simulink model "FusionMODEL_version1"  (R2018a)
settings: Solver=FixedStepAuto  StartTime=0.0  StopTime=SimulationTime  FixedStep=SamplingTime  RelTol=1e-3
undefined symbols (not defined in the file or in its folder): ACTIVATE_CAM, ACTIVATE_RAD, CAM1_detTimeStamp, CAM1_MeasNoise, CAM1_objClassID, CAM1_PX, CAM1_PY, CAM1_VX, CAM1_VY, CAM2_detTimeStamp, CAM2_MeasNoise, CAM2_objClassID, CAM2_PX, CAM2_PY, CAM2_VX, CAM2_VY, CAM3_detTimeStamp, CAM3_MeasNoise, CAM3_objClassID, CAM3_PX, CAM3_PY, CAM3_VX, CAM3_VY, CAM4_detTimeStamp, CAM4_MeasNoise, CAM4_objClassID, CAM4_PX, CAM4_PY, CAM4_VX, CAM4_VY, CAM5_detTimeStamp, CAM5_MeasNoise, CAM5_objClassID, CAM5_PX, CAM5_PY, CAM5_VX, CAM5_VY, CAM6_detTimeStamp, CAM6_MeasNoise, CAM6_objClassID, CAM6_PX, CAM6_PY, CAM6_VX, CAM6_VY, CAM7_detTimeStamp, CAM7_MeasNoise, CAM7_objClassID, CAM7_PX, CAM7_PY, CAM7_VX, CAM7_VY, CAM8_detTimeStamp, CAM8_MeasNoise, CAM8_objClassID, CAM8_PX, CAM8_PY, CAM8_VX, CAM8_VY, CAM_nMeas, CAM_TYPE ... (+151)
libraries: simulink_extras x2
(part 1 of 6)
settings Model: SimulationMode=accelerator  Creator=Udit Bhaskar  LastModifiedBy=Udit Bhaskar

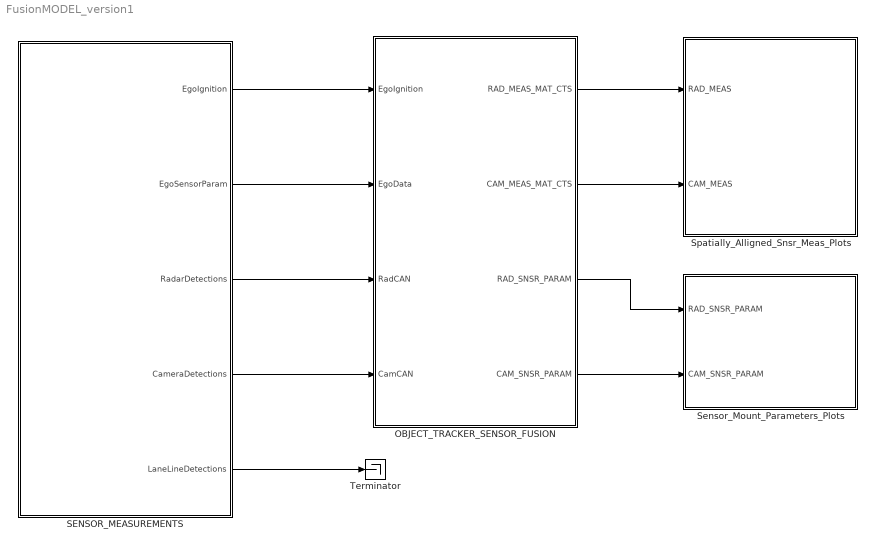
== system FusionMODEL_version1 ==
  OBJECT_TRACKER_SENSOR_FUSION : Subsystem
  SENSOR_MEASUREMENTS : Subsystem
  Sensor_Mount_Parameters_Plots : Subsystem
  Spatially_Alligned_Snsr_Meas_Plots : Subsystem
  Terminator : Terminator
  wires:
  SENSOR_MEASUREMENTS/5(LaneLineDetections) -> Terminator/1
  SENSOR_MEASUREMENTS/3(RadarDetections) -> OBJECT_TRACKER_SENSOR_FUSION/3(RadCAN)
  SENSOR_MEASUREMENTS/2(EgoSensorParam) -> OBJECT_TRACKER_SENSOR_FUSION/2(EgoData)
  SENSOR_MEASUREMENTS/4(CameraDetections) -> OBJECT_TRACKER_SENSOR_FUSION/4(CamCAN)
  SENSOR_MEASUREMENTS/1(EgoIgnition) -> OBJECT_TRACKER_SENSOR_FUSION/1(EgoIgnition)
  OBJECT_TRACKER_SENSOR_FUSION/1(RAD_MEAS_MAT_CTS) -> Spatially_Alligned_Snsr_Meas_Plots/1(RAD_MEAS)
  OBJECT_TRACKER_SENSOR_FUSION/2(CAM_MEAS_MAT_CTS) -> Spatially_Alligned_Snsr_Meas_Plots/2(CAM_MEAS)
  OBJECT_TRACKER_SENSOR_FUSION/3(RAD_SNSR_PARAM) -> Sensor_Mount_Parameters_Plots/1(RAD_SNSR_PARAM)
  OBJECT_TRACKER_SENSOR_FUSION/4(CAM_SNSR_PARAM) -> Sensor_Mount_Parameters_Plots/2(CAM_SNSR_PARAM)

== system FusionMODEL_version1/OBJECT_TRACKER_SENSOR_FUSION ==
  EgoIgnition : Inport
  EgoData : Inport  Port=2
  RadCAN : Inport  Port=3
  CamCAN : Inport  Port=4
  Ground1 : Ground
  Ground2 : Ground
  SET_SENSOR_CALLIBRATION_PARAMETER : Subsystem
  SPATIAL_ALLIGNMENT : Subsystem
  Terminator2 : Terminator
  Unit Delay : UnitDelay  InitialCondition=false  SampleTime=-1
  RAD_MEAS_MAT_CTS : Outport
  CAM_MEAS_MAT_CTS : Outport  Port=2
  RAD_SNSR_PARAM : Outport  Port=3
  CAM_SNSR_PARAM : Outport  Port=4
  wires:
  Ground2/1 -> SET_SENSOR_CALLIBRATION_PARAMETER/2(RADSnsrParam)
  SET_SENSOR_CALLIBRATION_PARAMETER/1(RadarCalibParamUpd) -> RAD_SNSR_PARAM/1, SPATIAL_ALLIGNMENT/1(RadarCallibrationParam)
  EgoData/1 -> Terminator2/1
  SPATIAL_ALLIGNMENT/1(RadarMeasTransformed) -> RAD_MEAS_MAT_CTS/1
  RadCAN/1 -> SPATIAL_ALLIGNMENT/3(RadarCAN)
  SPATIAL_ALLIGNMENT/2(CameraMeasTransformed) -> CAM_MEAS_MAT_CTS/1
  Ground1/1 -> SET_SENSOR_CALLIBRATION_PARAMETER/1(CamCalibParam)
  CamCAN/1 -> SPATIAL_ALLIGNMENT/4(CameraCAN)
  EgoIgnition/1 -> Unit Delay/1
  Unit Delay/1 -> SET_SENSOR_CALLIBRATION_PARAMETER/Trigger
  SET_SENSOR_CALLIBRATION_PARAMETER/2(CameraCalibParamUpd) -> CAM_SNSR_PARAM/1, SPATIAL_ALLIGNMENT/2(CameraCallibrationParam)

== system FusionMODEL_version1/SENSOR_MEASUREMENTS ==
  RADAR_CAMERA_EGO_SENSOR_INTERFACE : Subsystem
  Subsystem : Subsystem
  Subsystem1 : Subsystem
  EgoIgnition : Outport
  EgoSensorParam : Outport  Port=2
  RadarDetections : Outport  Port=3
  CameraDetections : Outport  Port=4
  LaneLineDetections : Outport  Port=5
  wires:
  RADAR_CAMERA_EGO_SENSOR_INTERFACE/11(C5) -> Subsystem/11(C5)
  RADAR_CAMERA_EGO_SENSOR_INTERFACE/4(R4) -> Subsystem/4(R4)
  RADAR_CAMERA_EGO_SENSOR_INTERFACE/2(R2) -> Subsystem/2(R2)
  RADAR_CAMERA_EGO_SENSOR_INTERFACE/5(R5) -> Subsystem/5(R5)
  RADAR_CAMERA_EGO_SENSOR_INTERFACE/6(R6) -> Subsystem/6(R6)
  RADAR_CAMERA_EGO_SENSOR_INTERFACE/1(R1) -> Subsystem/1(R1)
  Subsystem/1(RadarMeasurementCAN) -> RadarDetections/1
  RADAR_CAMERA_EGO_SENSOR_INTERFACE/9(C3) -> Subsystem/9(C3)
  RADAR_CAMERA_EGO_SENSOR_INTERFACE/8(C2) -> Subsystem/8(C2)
  RADAR_CAMERA_EGO_SENSOR_INTERFACE/3(R3) -> Subsystem/3(R3)
  RADAR_CAMERA_EGO_SENSOR_INTERFACE/13(C7) -> Subsystem/13(C7)
  RADAR_CAMERA_EGO_SENSOR_INTERFACE/7(C1) -> Subsystem/7(C1)
  RADAR_CAMERA_EGO_SENSOR_INTERFACE/10(C4) -> Subsystem/10(C4)
  RADAR_CAMERA_EGO_SENSOR_INTERFACE/12(C6) -> Subsystem/12(C6)
  Subsystem/2(CameraMeasurementCAN) -> CameraDetections/1
  RADAR_CAMERA_EGO_SENSOR_INTERFACE/14(C8) -> Subsystem/14(C8)
  RADAR_CAMERA_EGO_SENSOR_INTERFACE/15(CAM_LINE1) -> Subsystem1/1(CAM_LINE1)
  RADAR_CAMERA_EGO_SENSOR_INTERFACE/16(CAM_LINE2) -> Subsystem1/2(CAM_LINE2)
  RADAR_CAMERA_EGO_SENSOR_INTERFACE/17(CAM_LINE3) -> Subsystem1/3(CAM_LINE3)
  RADAR_CAMERA_EGO_SENSOR_INTERFACE/18(CAM_LINE4) -> Subsystem1/4(CAM_LINE4)
  RADAR_CAMERA_EGO_SENSOR_INTERFACE/19(CAM_LINE5) -> Subsystem1/5(CAM_LINE5)
  RADAR_CAMERA_EGO_SENSOR_INTERFACE/20(CAM_LINE6) -> Subsystem1/6(CAM_LINE6)
  RADAR_CAMERA_EGO_SENSOR_INTERFACE/21(CAM_LINE7) -> Subsystem1/7(CAM_LINE7)
  RADAR_CAMERA_EGO_SENSOR_INTERFACE/22(CAM_LINE8) -> Subsystem1/8(CAM_LINE8)
  Subsystem1/1(LineMeasurementsCAN) -> LaneLineDetections/1
  RADAR_CAMERA_EGO_SENSOR_INTERFACE/23(EGO) -> EgoSensorParam/1
  RADAR_CAMERA_EGO_SENSOR_INTERFACE/24(EgoIgnition) -> EgoIgnition/1

== system FusionMODEL_version1/Sensor_Mount_Parameters_Plots ==
  RAD_SNSR_PARAM : Inport
  CAM_SNSR_PARAM : Inport  Port=2
  CameraMountParametersPlots : Subsystem
  RadarMountParametersPlots : Subsystem
  wires:
  RAD_SNSR_PARAM/1 -> RadarMountParametersPlots/1(In1)
  CAM_SNSR_PARAM/1 -> CameraMountParametersPlots/1(In1)

== system FusionMODEL_version1/Spatially_Alligned_Snsr_Meas_Plots ==
  RAD_MEAS : Inport
  CAM_MEAS : Inport  Port=2
  Bus Selector : BusSelector  OutputSignals=MeasArray,ValidCumulativeMeasCount
  Bus Selector1 : BusSelector  OutputSignals=MeasArray,ValidCumulativeMeasCount
  CameraMeasCTS : Scope
  RadarMeasCTS : Scope
  Selector : Selector  NumberOfDimensions=2  InputPortWidth=3  IndexOptions=Select all,Index vector (port)  Indices=[1 3],1  OutputSizes=1,1
  Selector1 : Selector  NumberOfDimensions=2  InputPortWidth=3  IndexOptions=Index vector (dialog),Index vector (dialog)  Indices=1,1:30  OutputSizes=1,1
  Selector2 : Selector  NumberOfDimensions=2  InputPortWidth=3  IndexOptions=Select all,Index vector (port)  Indices=[1 3],1  OutputSizes=1,1
  Selector3 : Selector  NumberOfDimensions=2  InputPortWidth=3  IndexOptions=Index vector (dialog),Index vector (dialog)  Indices=1,1:30  OutputSizes=1,1
  Width : Width
  Width1 : Width
  nCameraMeasurements : Scope
  nRadarMeasurements : Scope
  wires:
  Bus Selector/1 -> Selector1/1  "<MeasArray>"
  Bus Selector/2 -> Selector/1, Width/1  "<ValidCumulativeMeasCount>"
  Width/1 -> Selector/2
  Selector1/1 -> RadarMeasCTS/1
  RAD_MEAS/1 -> Bus Selector/1
  Selector/1 -> nRadarMeasurements/1
  Bus Selector1/1 -> Selector3/1  "<MeasArray>"
  CAM_MEAS/1 -> Bus Selector1/1
  Width1/1 -> Selector2/2
  Selector2/1 -> nCameraMeasurements/1
  Selector3/1 -> CameraMeasCTS/1
  Bus Selector1/2 -> Selector2/1, Width1/1  "<ValidCumulativeMeasCount>"

== system FusionMODEL_version1/OBJECT_TRACKER_SENSOR_FUSION/SET_SENSOR_CALLIBRATION_PARAMETER ==
  CamCalibParam : Inport  OutDataTypeStr=Bus: CAM_SENSOR_PARAM  PortDimensions=nCameraActive  BusOutputAsStruct=on
  RADSnsrParam : Inport  Port=2  OutDataTypeStr=Bus: RAD_SENSOR_PARAM  PortDimensions=1
  Trigger : TriggerPort  VariantControl=Variant  PortDimensions=1
  SET_CAMERA_SENSOR_PARAM : Subsystem  TreatAsAtomicUnit=on
  SET_RADAR_SENSOR_PARAM : Subsystem
  RadarCalibParamUpd : Outport
  CameraCalibParamUpd : Outport  Port=2
  wires:
  SET_CAMERA_SENSOR_PARAM/1(CAMSnsrParamUpd) -> CameraCalibParamUpd/1
  CamCalibParam/1 -> SET_CAMERA_SENSOR_PARAM/1(CAMSnsrParam)
  RADSnsrParam/1 -> SET_RADAR_SENSOR_PARAM/1(RADSnsrParam)
  SET_RADAR_SENSOR_PARAM/1(RADSnsrParamUpd) -> RadarCalibParamUpd/1

== system FusionMODEL_version1/OBJECT_TRACKER_SENSOR_FUSION/SPATIAL_ALLIGNMENT ==
  RadarCallibrationParam : Inport
  CameraCallibrationParam : Inport  Port=2
  RadarCAN : Inport  Port=3
  CameraCAN : Inport  Port=4
  CAMERA_MEASUREMENTS_SPATIAL_ALLIGNMENT : Subsystem
  GET_CAM_MEAS : Subsystem
  GET_RAD_MEAS : Subsystem
  RADAR_MEASUREMENTS_SPATIAL_ALLIGNMENT : Subsystem
  RadarMeasTransformed : Outport
  CameraMeasTransformed : Outport  Port=2
  wires:
  RadarCAN/1 -> GET_RAD_MEAS/2(RadarMeas)
  CameraCAN/1 -> GET_CAM_MEAS/2(CameraMeas)
  GET_CAM_MEAS/2(<C1>) -> CAMERA_MEASUREMENTS_SPATIAL_ALLIGNMENT/2(C1)
  GET_CAM_MEAS/3(<C2>) -> CAMERA_MEASUREMENTS_SPATIAL_ALLIGNMENT/3(C2)
  GET_CAM_MEAS/4(<C3>) -> CAMERA_MEASUREMENTS_SPATIAL_ALLIGNMENT/4(C3)
  GET_CAM_MEAS/5(<C4>) -> CAMERA_MEASUREMENTS_SPATIAL_ALLIGNMENT/5(C4)
  GET_CAM_MEAS/6(<C5>) -> CAMERA_MEASUREMENTS_SPATIAL_ALLIGNMENT/6(C5)
  GET_CAM_MEAS/7(<C6>) -> CAMERA_MEASUREMENTS_SPATIAL_ALLIGNMENT/7(C6)
  GET_CAM_MEAS/8(<C7>) -> CAMERA_MEASUREMENTS_SPATIAL_ALLIGNMENT/8(C7)
  GET_CAM_MEAS/9(<C8>) -> CAMERA_MEASUREMENTS_SPATIAL_ALLIGNMENT/9(C8)
  GET_RAD_MEAS/2(<R1>) -> RADAR_MEASUREMENTS_SPATIAL_ALLIGNMENT/2(R1)
  GET_RAD_MEAS/3(<R2>) -> RADAR_MEASUREMENTS_SPATIAL_ALLIGNMENT/3(R2)
  GET_RAD_MEAS/4(<R3>) -> RADAR_MEASUREMENTS_SPATIAL_ALLIGNMENT/4(R3)
  GET_RAD_MEAS/5(<R4>) -> RADAR_MEASUREMENTS_SPATIAL_ALLIGNMENT/5(R4)
  GET_RAD_MEAS/6(<R5>) -> RADAR_MEASUREMENTS_SPATIAL_ALLIGNMENT/6(R5)
  GET_RAD_MEAS/7(<R6>) -> RADAR_MEASUREMENTS_SPATIAL_ALLIGNMENT/7(R6)
  GET_RAD_MEAS/1(SnsrParam) -> RADAR_MEASUREMENTS_SPATIAL_ALLIGNMENT/1(RadarCalibParam)
  RadarCallibrationParam/1 -> GET_RAD_MEAS/1(RadarParam)
  GET_CAM_MEAS/1(SnsrParam) -> CAMERA_MEASUREMENTS_SPATIAL_ALLIGNMENT/1(CameraCalibParam)
  CameraCallibrationParam/1 -> GET_CAM_MEAS/1(CameraParam)
  CAMERA_MEASUREMENTS_SPATIAL_ALLIGNMENT/1(CameraMeasTransformed) -> CameraMeasTransformed/1
  RADAR_MEASUREMENTS_SPATIAL_ALLIGNMENT/1(RadarMeasTransformed) -> RadarMeasTransformed/1

== system FusionMODEL_version1/SENSOR_MEASUREMENTS/RADAR_CAMERA_EGO_SENSOR_INTERFACE ==
  CameraSensors : Subsystem
  Clock : Subsystem
  EgoSensors : Subsystem
  Ground{,1..3} (4 alike) : Ground
  RadarSensors : Subsystem
  RoadSensors : Subsystem
  R1 : Outport
  R2 : Outport  Port=2
  R3 : Outport  Port=3
  R4 : Outport  Port=4
  R5 : Outport  Port=5
  R6 : Outport  Port=6
  C1 : Outport  Port=7
  C2 : Outport  Port=8
  C3 : Outport  Port=9
  C4 : Outport  Port=10
  C5 : Outport  Port=11
  C6 : Outport  Port=12
  C7 : Outport  Port=13
  C8 : Outport  Port=14
  CAM_LINE1 : Outport  Port=15
  CAM_LINE2 : Outport  Port=16
  CAM_LINE3 : Outport  Port=17
  CAM_LINE4 : Outport  Port=18
  CAM_LINE5 : Outport  Port=19
  CAM_LINE6 : Outport  Port=20
  CAM_LINE7 : Outport  Port=21
  CAM_LINE8 : Outport  Port=22
  EGO : Outport  Port=23
  EgoIgnition : Outport  Port=24
  wires:
  RadarSensors/6(R6) -> R6/1
  RadarSensors/4(R4) -> R4/1
  Clock/2(nObjRadar) -> RadarSensors/2(nObjRadar)
  Clock/3(nObjCamera) -> CameraSensors/2(nObjCamera)
  CameraSensors/3(C3) -> C3/1
  RadarSensors/5(R5) -> R5/1
  CameraSensors/5(C5) -> C5/1
  CameraSensors/4(C4) -> C4/1
  CameraSensors/8(C8) -> C8/1
  CameraSensors/7(C7) -> C7/1
  CameraSensors/6(C6) -> C6/1
  CameraSensors/2(C2) -> C2/1
  RadarSensors/2(R2) -> R2/1
  RadarSensors/3(R3) -> R3/1
  CameraSensors/1(C1) -> C1/1
  RadarSensors/1(R1) -> R1/1
  Clock/1(time) -> CameraSensors/1(time), RoadSensors/1(time), EgoSensors/1(timeIdx), RadarSensors/1(time)
  Clock/4(nLinesCamera) -> RoadSensors/2(nLinesCamera)
  RoadSensors/1(C1) -> CAM_LINE1/1
  RoadSensors/2(C2) -> CAM_LINE2/1
  RoadSensors/3(C3) -> CAM_LINE3/1
  RoadSensors/4(C4) -> CAM_LINE4/1
  RoadSensors/5(C5) -> CAM_LINE5/1
  RoadSensors/6(C6) -> CAM_LINE6/1
  RoadSensors/7(C7) -> CAM_LINE7/1
  RoadSensors/8(C8) -> CAM_LINE8/1
  EgoSensors/1(EgoSensorData) -> EGO/1
  Ground1/1 -> RadarSensors/3(RADSensorBUS)
  Ground2/1 -> CameraSensors/3(CAMSensorBUS)
  Ground/1 -> EgoSensors/2(In1)
  Ground3/1 -> RoadSensors/3(CameraLineCoeff1)
  EgoSensors/2(EgoIgnitionStatus) -> EgoIgnition/1

== system FusionMODEL_version1/SENSOR_MEASUREMENTS/Subsystem ==
  R1 : Inport
  R2 : Inport  Port=2
  R3 : Inport  Port=3
  R4 : Inport  Port=4
  R5 : Inport  Port=5
  R6 : Inport  Port=6
  C1 : Inport  Port=7
  C2 : Inport  Port=8
  C3 : Inport  Port=9
  C4 : Inport  Port=10
  C5 : Inport  Port=11
  C6 : Inport  Port=12
  C7 : Inport  Port=13
  C8 : Inport  Port=14
  Bus Creator : BusCreator  Inputs=6  OutDataTypeStr=Bus: RAD_MEAS_INTERFACE  NonVirtualBus=on
  Bus Creator1 : BusCreator  Inputs=8  OutDataTypeStr=Bus: CAM_MEAS_INTERFACE  NonVirtualBus=on
  RadarMeasurementCAN : Outport
  CameraMeasurementCAN : Outport  Port=2
  wires:
  R1/1 -> Bus Creator/1  "R1"
  R6/1 -> Bus Creator/6  "R6"
  R5/1 -> Bus Creator/5  "R5"
  R4/1 -> Bus Creator/4  "R4"
  R3/1 -> Bus Creator/3  "R3"
  R2/1 -> Bus Creator/2  "R2"
  Bus Creator/1 -> RadarMeasurementCAN/1
  C1/1 -> Bus Creator1/1  "C1"
  C2/1 -> Bus Creator1/2  "C2"
  C3/1 -> Bus Creator1/3  "C3"
  C4/1 -> Bus Creator1/4  "C4"
  C5/1 -> Bus Creator1/5  "C5"
  C6/1 -> Bus Creator1/6  "C6"
  C7/1 -> Bus Creator1/7  "C7"
  C8/1 -> Bus Creator1/8  "C8"
  Bus Creator1/1 -> CameraMeasurementCAN/1

== system FusionMODEL_version1/SENSOR_MEASUREMENTS/Subsystem1 ==
  CAM_LINE1 : Inport
  CAM_LINE2 : Inport  Port=2
  CAM_LINE3 : Inport  Port=3
  CAM_LINE4 : Inport  Port=4
  CAM_LINE5 : Inport  Port=5
  CAM_LINE6 : Inport  Port=6
  CAM_LINE7 : Inport  Port=7
  CAM_LINE8 : Inport  Port=8
  Bus Creator : BusCreator  Inputs=8  OutDataTypeStr=Bus: LINE_MEAS_INTERFACE  NonVirtualBus=on
  LineMeasurementsCAN : Outport
  wires:
  CAM_LINE1/1 -> Bus Creator/1  "C1_LINE"
  CAM_LINE2/1 -> Bus Creator/2  "C2_LINE"
  CAM_LINE3/1 -> Bus Creator/3  "C3_LINE"
  CAM_LINE4/1 -> Bus Creator/4  "C4_LINE"
  CAM_LINE5/1 -> Bus Creator/5  "C5_LINE"
  CAM_LINE6/1 -> Bus Creator/6  "C6_LINE"
  CAM_LINE7/1 -> Bus Creator/7  "C7_LINE"
  CAM_LINE8/1 -> Bus Creator/8  "C8_LINE"
  Bus Creator/1 -> LineMeasurementsCAN/1

== system FusionMODEL_version1/Sensor_Mount_Parameters_Plots/CameraMountParametersPlots ==
  In1 : Inport
  Bus Selector{,1..2,4,9,11,14,16} (8 alike) : BusSelector  OutputSignals=CameraID,isActive,MountX,MountY,MountYaw,nMeas,CameraType
  Bus Selector{3,5,7..8,10,12..13,15} (8 alike) : BusSelector  OutputSignals=MaxRange
  Bus Selector6 : BusSelector  OutputSignals=signal2,signal1
  Scope{,1..7} (8 alike) : Scope  NumInputPorts=8
  Selector : Selector  NumberOfDimensions=2  InputPortWidth=3  IndexOptions=Select all,Index vector (dialog)  Indices=[1 3],1  OutputSizes=1,1
  Selector1 : Selector  NumberOfDimensions=2  InputPortWidth=3  IndexOptions=Select all,Index vector (dialog)  Indices=[1 3],2  OutputSizes=1,1
  Selector{6..13} (8 alike) : Selector  NumberOfDimensions=2  InputPortWidth=3  IndexOptions=Select all,Index vector (port)  Indices=[1 3],1  OutputSizes=1,1
  Selector14 : Selector  NumberOfDimensions=2  InputPortWidth=3  IndexOptions=Select all,Index vector (dialog)  Indices=[1 3],7  OutputSizes=1,1
  Selector15 : Selector  NumberOfDimensions=2  InputPortWidth=3  IndexOptions=Select all,Index vector (dialog)  Indices=[1 3],8  OutputSizes=1,1
  Selector2 : Selector  NumberOfDimensions=2  InputPortWidth=3  IndexOptions=Select all,Index vector (dialog)  Indices=[1 3],3  OutputSizes=1,1
  Selector3 : Selector  NumberOfDimensions=2  InputPortWidth=3  IndexOptions=Select all,Index vector (dialog)  Indices=[1 3],4  OutputSizes=1,1
  Selector4 : Selector  NumberOfDimensions=2  InputPortWidth=3  IndexOptions=Select all,Index vector (dialog)  Indices=[1 3],5  OutputSizes=1,1
  Selector5 : Selector  NumberOfDimensions=2  InputPortWidth=3  IndexOptions=Select all,Index vector (dialog)  Indices=[1 3],6  OutputSizes=1,1
  wires:
  Selector/1 -> Bus Selector/1
  Bus Selector/1 -> Scope/1  "<CameraID>"
  Bus Selector/2 -> Scope/2  "<isActive>"
  Bus Selector/3 -> Scope/3  "<MountX>"
  Bus Selector/4 -> Scope/4  "<MountY>"
  Bus Selector/5 -> Scope/5  "<MountYaw>"
  Bus Selector/6 -> Scope/6  "<nMeas>"
  Bus Selector/7 -> Selector6/2, Scope/7  "<CameraType>"
  Selector6/1 -> Bus Selector7/1
  Bus Selector7/1 -> Scope/8  "<MaxRange>"
  Selector1/1 -> Bus Selector1/1
  Bus Selector1/1 -> Scope6/1  "<CameraID>"
  Bus Selector1/2 -> Scope6/2  "<isActive>"
  Bus Selector1/3 -> Scope6/3  "<MountX>"
  Bus Selector1/4 -> Scope6/4  "<MountY>"
  Bus Selector1/5 -> Scope6/5  "<MountYaw>"
  Bus Selector1/6 -> Scope6/6  "<nMeas>"
  Bus Selector1/7 -> Selector7/2, Scope6/7  "<CameraType>"
  Bus Selector8/1 -> Scope6/8  "<MaxRange>"
  Selector7/1 -> Bus Selector8/1
  Selector8/1 -> Bus Selector3/1
  Bus Selector2/4 -> Scope2/4  "<MountY>"
  Bus Selector2/5 -> Scope2/5  "<MountYaw>"
  Bus Selector2/1 -> Scope2/1  "<CameraID>"
  Bus Selector3/1 -> Scope2/8  "<MaxRange>"
  Bus Selector2/2 -> Scope2/2  "<isActive>"
  Bus Selector2/3 -> Scope2/3  "<MountX>"
  Bus Selector2/7 -> Selector8/2, Scope2/7  "<CameraType>"
  Bus Selector2/6 -> Scope2/6  "<nMeas>"
  Selector2/1 -> Bus Selector2/1
  Selector9/1 -> Bus Selector5/1
  Bus Selector4/4 -> Scope3/4  "<MountY>"
  Bus Selector4/5 -> Scope3/5  "<MountYaw>"
  Bus Selector4/1 -> Scope3/1  "<CameraID>"
  Bus Selector5/1 -> Scope3/8  "<MaxRange>"
  Bus Selector4/2 -> Scope3/2  "<isActive>"
  Bus Selector4/3 -> Scope3/3  "<MountX>"
  Bus Selector4/7 -> Selector9/2, Scope3/7  "<CameraType>"
  Bus Selector4/6 -> Scope3/6  "<nMeas>"
  Selector3/1 -> Bus Selector4/1
  Selector10/1 -> Bus Selector10/1
  Bus Selector9/4 -> Scope4/4  "<MountY>"
  Bus Selector9/5 -> Scope4/5  "<MountYaw>"
  Bus Selector9/1 -> Scope4/1  "<CameraID>"
  Bus Selector10/1 -> Scope4/8  "<MaxRange>"
  Bus Selector9/2 -> Scope4/2  "<isActive>"
  Bus Selector9/3 -> Scope4/3  "<MountX>"
  Bus Selector9/7 -> Selector10/2, Scope4/7  "<CameraType>"
  Bus Selector9/6 -> Scope4/6  "<nMeas>"
  Selector4/1 -> Bus Selector9/1
  Selector11/1 -> Bus Selector12/1
  Bus Selector11/4 -> Scope5/4  "<MountY>"
  Bus Selector11/5 -> Scope5/5  "<MountYaw>"
  Bus Selector11/1 -> Scope5/1  "<CameraID>"
  Bus Selector12/1 -> Scope5/8  "<MaxRange>"
  Bus Selector11/2 -> Scope5/2  "<isActive>"
  Bus Selector11/3 -> Scope5/3  "<MountX>"
  Bus Selector11/7 -> Selector11/2, Scope5/7  "<CameraType>"
  Bus Selector11/6 -> Scope5/6  "<nMeas>"
  Selector5/1 -> Bus Selector11/1
  In1/1 -> Bus Selector6/1
  Bus Selector6/2 -> Selector12/1, Selector13/1, Selector11/1, Selector10/1, Selector9/1, Selector8/1, Selector7/1, Selector6/1  "<signal1>"
  Selector15/1 -> Bus Selector14/1
  Bus Selector16/2 -> Scope1/2  "<isActive>"
  Bus Selector13/1 -> Scope1/8  "<MaxRange>"
  Bus Selector16/1 -> Scope1/1  "<CameraID>"
  Bus Selector14/6 -> Scope7/6  "<nMeas>"
  Bus Selector14/5 -> Scope7/5  "<MountYaw>"
  Bus Selector14/3 -> Scope7/3  "<MountX>"
  Bus Selector16/7 -> Selector12/2, Scope1/7  "<CameraType>"
  Selector14/1 -> Bus Selector16/1
  Bus Selector14/7 -> Selector13/2, Scope7/7  "<CameraType>"
  Bus Selector14/2 -> Scope7/2  "<isActive>"
  Bus Selector15/1 -> Scope7/8  "<MaxRange>"
  Selector12/1 -> Bus Selector13/1
  Bus Selector16/5 -> Scope1/5  "<MountYaw>"
  Bus Selector16/3 -> Scope1/3  "<MountX>"
  Bus Selector16/4 -> Scope1/4  "<MountY>"
  Bus Selector6/1 -> Selector14/1, Selector15/1, Selector5/1, Selector4/1, Selector3/1, Selector2/1, Selector1/1, Selector/1  "<signal2>"
  Bus Selector16/6 -> Scope1/6  "<nMeas>"
  Bus Selector14/1 -> Scope7/1  "<CameraID>"
  Bus Selector14/4 -> Scope7/4  "<MountY>"
  Selector13/1 -> Bus Selector15/1

== system FusionMODEL_version1/Sensor_Mount_Parameters_Plots/RadarMountParametersPlots ==
  In1 : Inport
  Bus Selector{,1..2,4,9,11} (6 alike) : BusSelector  OutputSignals=RadarID,isActive,MountX,MountY,MountYaw,nMeas,RadarType
  Bus Selector{3,5,7..8,10,12} (6 alike) : BusSelector  OutputSignals=MaxRange
  Bus Selector6 : BusSelector  OutputSignals=RadarExtrinsics,RadarIntrinsics
  Scope{,2..6} (6 alike) : Scope  NumInputPorts=8
  Selector : Selector  NumberOfDimensions=2  InputPortWidth=3  IndexOptions=Select all,Index vector (dialog)  Indices=[1 3],1  OutputSizes=1,1
  Selector1 : Selector  NumberOfDimensions=2  InputPortWidth=3  IndexOptions=Select all,Index vector (dialog)  Indices=[1 3],2  OutputSizes=1,1
  Selector{6..11} (6 alike) : Selector  NumberOfDimensions=2  InputPortWidth=3  IndexOptions=Select all,Index vector (port)  Indices=[1 3],1  OutputSizes=1,1
  Selector2 : Selector  NumberOfDimensions=2  InputPortWidth=3  IndexOptions=Select all,Index vector (dialog)  Indices=[1 3],3  OutputSizes=1,1
  Selector3 : Selector  NumberOfDimensions=2  InputPortWidth=3  IndexOptions=Select all,Index vector (dialog)  Indices=[1 3],4  OutputSizes=1,1
  Selector4 : Selector  NumberOfDimensions=2  InputPortWidth=3  IndexOptions=Select all,Index vector (dialog)  Indices=[1 3],5  OutputSizes=1,1
  Selector5 : Selector  NumberOfDimensions=2  InputPortWidth=3  IndexOptions=Select all,Index vector (dialog)  Indices=[1 3],6  OutputSizes=1,1
  wires:
  Selector/1 -> Bus Selector/1
  In1/1 -> Bus Selector6/1
  Bus Selector6/1 -> Selector/1, Selector5/1, Selector4/1, Selector3/1, Selector2/1, Selector1/1  "<RadarExtrinsics>"
  Bus Selector/1 -> Scope/1  "<RadarID>"
  Bus Selector/2 -> Scope/2  "<isActive>"
  Bus Selector/3 -> Scope/3  "<MountX>"
  Bus Selector/4 -> Scope/4  "<MountY>"
  Bus Selector/5 -> Scope/5  "<MountYaw>"
  Bus Selector/6 -> Scope/6  "<nMeas>"
  Bus Selector/7 -> Selector6/2, Scope/7  "<RadarType>"
  Selector6/1 -> Bus Selector7/1
  Bus Selector7/1 -> Scope/8  "<MaxRange>"
  Selector1/1 -> Bus Selector1/1
  Bus Selector1/1 -> Scope6/1  "<RadarID>"
  Bus Selector1/2 -> Scope6/2  "<isActive>"
  Bus Selector1/3 -> Scope6/3  "<MountX>"
  Bus Selector1/4 -> Scope6/4  "<MountY>"
  Bus Selector1/5 -> Scope6/5  "<MountYaw>"
  Bus Selector1/6 -> Scope6/6  "<nMeas>"
  Bus Selector1/7 -> Selector7/2, Scope6/7  "<RadarType>"
  Bus Selector8/1 -> Scope6/8  "<MaxRange>"
  Selector7/1 -> Bus Selector8/1
  Selector8/1 -> Bus Selector3/1
  Bus Selector2/4 -> Scope2/4  "<MountY>"
  Bus Selector2/5 -> Scope2/5  "<MountYaw>"
  Bus Selector2/1 -> Scope2/1  "<RadarID>"
  Bus Selector3/1 -> Scope2/8  "<MaxRange>"
  Bus Selector2/2 -> Scope2/2  "<isActive>"
  Bus Selector2/3 -> Scope2/3  "<MountX>"
  Bus Selector2/7 -> Selector8/2, Scope2/7  "<RadarType>"
  Bus Selector2/6 -> Scope2/6  "<nMeas>"
  Selector2/1 -> Bus Selector2/1
  Selector9/1 -> Bus Selector5/1
  Bus Selector4/4 -> Scope3/4  "<MountY>"
  Bus Selector4/5 -> Scope3/5  "<MountYaw>"
  Bus Selector4/1 -> Scope3/1  "<RadarID>"
  Bus Selector5/1 -> Scope3/8  "<MaxRange>"
  Bus Selector4/2 -> Scope3/2  "<isActive>"
  Bus Selector4/3 -> Scope3/3  "<MountX>"
  Bus Selector4/7 -> Selector9/2, Scope3/7  "<RadarType>"
  Bus Selector4/6 -> Scope3/6  "<nMeas>"
  Selector3/1 -> Bus Selector4/1
  Selector10/1 -> Bus Selector10/1
  Bus Selector9/4 -> Scope4/4  "<MountY>"
  Bus Selector9/5 -> Scope4/5  "<MountYaw>"
  Bus Selector9/1 -> Scope4/1  "<RadarID>"
  Bus Selector10/1 -> Scope4/8  "<MaxRange>"
  Bus Selector9/2 -> Scope4/2  "<isActive>"
  Bus Selector9/3 -> Scope4/3  "<MountX>"
  Bus Selector9/7 -> Selector10/2, Scope4/7  "<RadarType>"
  Bus Selector9/6 -> Scope4/6  "<nMeas>"
  Selector4/1 -> Bus Selector9/1
  Selector11/1 -> Bus Selector12/1
  Bus Selector11/4 -> Scope5/4  "<MountY>"
  Bus Selector6/2 -> Selector11/1, Selector10/1, Selector9/1, Selector8/1, Selector7/1, Selector6/1  "<RadarIntrinsics>"
  Bus Selector11/5 -> Scope5/5  "<MountYaw>"
  Bus Selector11/1 -> Scope5/1  "<RadarID>"
  Bus Selector12/1 -> Scope5/8  "<MaxRange>"
  Bus Selector11/2 -> Scope5/2  "<isActive>"
  Bus Selector11/3 -> Scope5/3  "<MountX>"
  Bus Selector11/7 -> Selector11/2, Scope5/7  "<RadarType>"
  Bus Selector11/6 -> Scope5/6  "<nMeas>"
  Selector5/1 -> Bus Selector11/1

== system FusionMODEL_version1/OBJECT_TRACKER_SENSOR_FUSION/SET_SENSOR_CALLIBRATION_PARAMETER/SET_CAMERA_SENSOR_PARAM ==
  CAMSnsrParam : Inport
  GET_DATA : Subsystem
  SET_CAMERA_EXTRINSIC_PARAM : Subsystem  TreatAsAtomicUnit=on
  SET_CAMERA_INTRINSIC_PARAM : Subsystem  TreatAsAtomicUnit=on
  SET_DATA : Subsystem
  CAMSnsrParamUpd : Outport
  wires:
  SET_DATA/1(CAMSnsrParamUpd) -> CAMSnsrParamUpd/1
  CAMSnsrParam/1 -> GET_DATA/1(CAMSnsrParam)
  GET_DATA/2(CameraExtrinsics) -> SET_CAMERA_EXTRINSIC_PARAM/1(CameraCalibParam)
  GET_DATA/1(CameraIntrinsics) -> SET_CAMERA_INTRINSIC_PARAM/1(CameraCalibParam)
  SET_CAMERA_INTRINSIC_PARAM/1(CameraCalibParamSet) -> SET_DATA/1(CameraIntrinsics)
  SET_CAMERA_EXTRINSIC_PARAM/1(CameraCalibParamSet) -> SET_DATA/2(CameraExtrinsics)

== system FusionMODEL_version1/OBJECT_TRACKER_SENSOR_FUSION/SET_SENSOR_CALLIBRATION_PARAMETER/SET_RADAR_SENSOR_PARAM ==
  RADSnsrParam : Inport
  GET_DATA : Subsystem
  SET_DATA : Subsystem
  SET_RADAR_EXTRINSIC_PARAM : Subsystem  TreatAsAtomicUnit=on
  SET_RADAR_INTRINSIC_PARAM : Subsystem  TreatAsAtomicUnit=on
  RADSnsrParamUpd : Outport
  wires:
  RADSnsrParam/1 -> GET_DATA/1(RADSnsrParam)
  SET_DATA/1(RADSnsrParamUpd) -> RADSnsrParamUpd/1
  GET_DATA/2(<RadarExtrinsics>) -> SET_RADAR_EXTRINSIC_PARAM/1(RadarCalibParam)
  SET_RADAR_EXTRINSIC_PARAM/1(RadarCalibParamSet) -> SET_DATA/2(RadarExtrinsics)  "RadarIntrinsics"
  GET_DATA/1(<RadarIntrinsics>) -> SET_RADAR_INTRINSIC_PARAM/1(RadarCalibParam)
  SET_RADAR_INTRINSIC_PARAM/1(RadarCalibParamSet) -> SET_DATA/1(RadarIntrinsics)  "RadarExtrinsics"

== system FusionMODEL_version1/OBJECT_TRACKER_SENSOR_FUSION/SPATIAL_ALLIGNMENT/CAMERA_MEASUREMENTS_SPATIAL_ALLIGNMENT ==
  CameraCalibParam : Inport  BusOutputAsStruct=on
  C1 : Inport  Port=2
  C2 : Inport  Port=3
  C3 : Inport  Port=4
  C4 : Inport  Port=5
  C5 : Inport  Port=6
  C6 : Inport  Port=7
  C7 : Inport  Port=8
  C8 : Inport  Port=9
  For Iterator Subsystem : Subsystem  TreatAsAtomicUnit=on
  RadarMeasurementIndexes2 : Subsystem
  StartingIndexes1 : Subsystem
  CameraMeasTransformed : Outport
  wires:
  CameraCalibParam/1 -> For Iterator Subsystem/1(CameraCallibrationParam), StartingIndexes1/1(SnsrCallib)
  C6/1 -> For Iterator Subsystem/8(C6)
  C3/1 -> For Iterator Subsystem/5(C3)
  C4/1 -> For Iterator Subsystem/6(C4)
  C2/1 -> For Iterator Subsystem/4(C2)
  C1/1 -> For Iterator Subsystem/3(C1)
  StartingIndexes1/1(StartingIndexes) -> For Iterator Subsystem/2(RadarStartingIdx)
  C5/1 -> For Iterator Subsystem/7(C5)
  C7/1 -> For Iterator Subsystem/9(C7)
  C8/1 -> For Iterator Subsystem/10(C8)
  For Iterator Subsystem/2(CameraMeasTransformed) -> RadarMeasurementIndexes2/2(CTSmeasMAT)
  RadarMeasurementIndexes2/1(CTSmeasMATout) -> CameraMeasTransformed/1
  For Iterator Subsystem/4(CameraMeasRef) -> RadarMeasurementIndexes2/4(CTSRefMAT)
  For Iterator Subsystem/3(CameraMeasCOVTransformed) -> RadarMeasurementIndexes2/3(CTSCovMAT)
  For Iterator Subsystem/1(MaxNoValidMeas) -> RadarMeasurementIndexes2/1(validMeasCount)

== system FusionMODEL_version1/OBJECT_TRACKER_SENSOR_FUSION/SPATIAL_ALLIGNMENT/GET_CAM_MEAS ==
  CameraParam : Inport
  CameraMeas : Inport  Port=2
  Bus Selector1 : BusSelector  OutputSignals=C1,C2,C3,C4,C5,C6,C7,C8
  Bus Selector2 : BusSelector  OutputSignals=signal2
  SnsrParam : Outport
  <C1> : Outport  Port=2
  <C2> : Outport  Port=3
  <C3> : Outport  Port=4
  <C4> : Outport  Port=5
  <C5> : Outport  Port=6
  <C6> : Outport  Port=7
  <C7> : Outport  Port=8
  <C8> : Outport  Port=9
  wires:
  Bus Selector1/4 -> <C4>/1  "<C4>"
  Bus Selector1/6 -> <C6>/1  "<C6>"
  Bus Selector1/5 -> <C5>/1  "<C5>"
  CameraMeas/1 -> Bus Selector1/1
  Bus Selector1/1 -> <C1>/1  "<C1>"
  Bus Selector1/7 -> <C7>/1  "<C7>"
  Bus Selector1/8 -> <C8>/1  "<C8>"
  Bus Selector1/2 -> <C2>/1  "<C2>"
  Bus Selector1/3 -> <C3>/1  "<C3>"
  CameraParam/1 -> Bus Selector2/1
  Bus Selector2/1 -> SnsrParam/1  "<signal2>"

== system FusionMODEL_version1/OBJECT_TRACKER_SENSOR_FUSION/SPATIAL_ALLIGNMENT/GET_RAD_MEAS ==
  RadarParam : Inport
  RadarMeas : Inport  Port=2
  Bus Selector : BusSelector  OutputSignals=R1,R2,R3,R4,R5,R6
  Bus Selector1 : BusSelector  OutputSignals=RadarExtrinsics
  SnsrParam : Outport
  <R1> : Outport  Port=2
  <R2> : Outport  Port=3
  <R3> : Outport  Port=4
  <R4> : Outport  Port=5
  <R5> : Outport  Port=6
  <R6> : Outport  Port=7
  wires:
  Bus Selector/1 -> <R1>/1  "<R1>"
  Bus Selector/2 -> <R2>/1  "<R2>"
  Bus Selector/3 -> <R3>/1  "<R3>"
  Bus Selector/6 -> <R6>/1  "<R6>"
  Bus Selector/4 -> <R4>/1  "<R4>"
  Bus Selector/5 -> <R5>/1  "<R5>"
  RadarMeas/1 -> Bus Selector/1
  Bus Selector1/1 -> SnsrParam/1  "<RadarExtrinsics>"
  RadarParam/1 -> Bus Selector1/1

== system FusionMODEL_version1/OBJECT_TRACKER_SENSOR_FUSION/SPATIAL_ALLIGNMENT/RADAR_MEASUREMENTS_SPATIAL_ALLIGNMENT ==
  RadarCalibParam : Inport  BusOutputAsStruct=on
  R1 : Inport  Port=2
  R2 : Inport  Port=3
  R3 : Inport  Port=4
  R4 : Inport  Port=5
  R5 : Inport  Port=6
  R6 : Inport  Port=7
  RADAR_MEASUREMENTS_SPATIAL_ALLIGNMENT : Subsystem  TreatAsAtomicUnit=on
  SET_MEASUREMENTS : Subsystem
  StartingIndexes1 : Subsystem
  RadarMeasTransformed : Outport
  wires:
  StartingIndexes1/1(StartingIndexes) -> RADAR_MEASUREMENTS_SPATIAL_ALLIGNMENT/2(RadarStartingIdx)
  R1/1 -> RADAR_MEASUREMENTS_SPATIAL_ALLIGNMENT/3(R1)
  R2/1 -> RADAR_MEASUREMENTS_SPATIAL_ALLIGNMENT/4(R2)
  R4/1 -> RADAR_MEASUREMENTS_SPATIAL_ALLIGNMENT/6(R4)
  R5/1 -> RADAR_MEASUREMENTS_SPATIAL_ALLIGNMENT/7(R5)
  RadarCalibParam/1 -> RADAR_MEASUREMENTS_SPATIAL_ALLIGNMENT/1(RadarCallibrationParam), StartingIndexes1/1(SnsrCallib)
  R6/1 -> RADAR_MEASUREMENTS_SPATIAL_ALLIGNMENT/8(R6)
  R3/1 -> RADAR_MEASUREMENTS_SPATIAL_ALLIGNMENT/5(R3)
  RADAR_MEASUREMENTS_SPATIAL_ALLIGNMENT/1(RadarMeasTransformed) -> SET_MEASUREMENTS/1(CTSmeasMAT)
  RADAR_MEASUREMENTS_SPATIAL_ALLIGNMENT/4(MaxNoValidMeas) -> SET_MEASUREMENTS/4(validMeasCount)
  SET_MEASUREMENTS/1(CTSmeasMATout) -> RadarMeasTransformed/1
  RADAR_MEASUREMENTS_SPATIAL_ALLIGNMENT/2(RadarMeasCOVTransformed) -> SET_MEASUREMENTS/2(CTSCovMAT)
  RADAR_MEASUREMENTS_SPATIAL_ALLIGNMENT/3(RadarMeasRef) -> SET_MEASUREMENTS/3(CTSRefMAT)

== system FusionMODEL_version1/SENSOR_MEASUREMENTS/RADAR_CAMERA_EGO_SENSOR_INTERFACE/CameraSensors ==
  time : Inport
  nObjCamera : Inport  Port=2
  CAMSensorBUS : Inport  Port=3  OutDataTypeStr=Bus: CameraMeasParam  PortDimensions=200  BusOutputAsStruct=on
  Camera1 : Subsystem  TreatAsAtomicUnit=on
  Camera2 : Subsystem  TreatAsAtomicUnit=on
  Camera3 : Subsystem  TreatAsAtomicUnit=on
  Camera4 : Subsystem  TreatAsAtomicUnit=on
  Camera5 : Subsystem  TreatAsAtomicUnit=on
  Camera6 : Subsystem  TreatAsAtomicUnit=on
  Camera7 : Subsystem  TreatAsAtomicUnit=on
  Camera8 : Subsystem  TreatAsAtomicUnit=on
  C1 : Outport
  C2 : Outport  Port=2
  C3 : Outport  Port=3
  C4 : Outport  Port=4
  C5 : Outport  Port=5
  C6 : Outport  Port=6
  C7 : Outport  Port=7
  C8 : Outport  Port=8
  wires:
  CAMSensorBUS/1 -> Camera1/3(SensorMeas), Camera2/3(SensorMeas), Camera3/3(SensorMeas), Camera4/3(SensorMeas), Camera6/3(SensorMeas), Camera8/3(SensorMeas), Camera7/3(SensorMeas), Camera5/3(SensorMeas)
  nObjCamera/1 -> Camera4/2(nObjCamera), Camera6/2(nObjCamera), Camera8/2(nObjCamera), Camera7/2(nObjCamera), Camera5/2(nObjCamera), Camera3/2(nObjCamera), Camera2/2(nObjCamera), Camera1/2(nObjCamera)
  Camera1/1(C1) -> C1/1
  time/1 -> Camera1/1(timeIdx), Camera4/1(timeIdx), Camera5/1(timeIdx), Camera6/1(timeIdx), Camera8/1(timeIdx), Camera7/1(timeIdx), Camera3/1(timeIdx), Camera2/1(timeIdx)
  Camera4/1(C4) -> C4/1
  Camera3/1(C3) -> C3/1
  Camera6/1(C6) -> C6/1
  Camera5/1(C5) -> C5/1
  Camera2/1(C2) -> C2/1
  Camera7/1(C7) -> C7/1
  Camera8/1(C8) -> C8/1

== system FusionMODEL_version1/SENSOR_MEASUREMENTS/RADAR_CAMERA_EGO_SENSOR_INTERFACE/Clock ==
  note: A n Array Of maximum number of sensor measurements for each Radar
  note: A n Array Of maximum number of sensor measurements for each Camera
  Add : Sum
  Constant : Constant
  Constant1 : Constant  Value=RAD_nMeas
  Constant2 : Constant  Value=CAM_nMeas
  Constant3 : Constant  Value=int32([2, 2, 2, 2, 2, 2, 2, 2])
  Data Type Conversion : DataTypeConversion  OutDataTypeStr=int16
  Digital Clock : DigitalClock  SampleTime=-1
  Gain : Gain  Gain=1/SamplingTime
  time : Outport
  nObjRadar : Outport  Port=2
  nObjCamera : Outport  Port=3
  nLinesCamera : Outport  Port=4
  wires:
  Digital Clock/1 -> Gain/1
  Gain/1 -> Add/1
  Add/1 -> Data Type Conversion/1
  Constant/1 -> Add/2
  Data Type Conversion/1 -> time/1
  Constant1/1 -> nObjRadar/1
  Constant2/1 -> nObjCamera/1
  Constant3/1 -> nLinesCamera/1

== system FusionMODEL_version1/SENSOR_MEASUREMENTS/RADAR_CAMERA_EGO_SENSOR_INTERFACE/EgoSensors ==
  timeIdx : Inport
  In1 : Inport  Port=2  OutDataTypeStr=Bus: EGO_PARAM  PortDimensions=1
  Assignment : Assignment  DiagnosticForDimensions=Warning  IndexOptions=Index vector (dialog)  Indices=1  OutputSizes=1
  Bus Creator : BusCreator  Inputs=7  OutDataTypeStr=Bus: EGO_PARAM  NonVirtualBus=on
  ExtractMeasParam : Subsystem
  EgoSensorData : Outport
  EgoIgnitionStatus : Outport  Port=2
  wires:
  timeIdx/1 -> ExtractMeasParam/1(timeIdx)
  Bus Creator/1 -> Assignment/2
  Assignment/1 -> EgoSensorData/1
  ExtractMeasParam/1(EgoTimeStamp) -> Bus Creator/1  "TimeStamp"
  ExtractMeasParam/2(EgoPx) -> Bus Creator/2  "px"
  ExtractMeasParam/3(EgoPy) -> Bus Creator/3  "py"
  ExtractMeasParam/4(EgoVx) -> Bus Creator/4  "vx"
  ExtractMeasParam/6(EgoYaw) -> Bus Creator/6  "yaw"
  ExtractMeasParam/7(EgoYawRate) -> Bus Creator/7  "yawRate"
  ExtractMeasParam/5(EgoVy) -> Bus Creator/5  "vy"
  In1/1 -> Assignment/1
  ExtractMeasParam/8(EgoIgnitionStatus) -> EgoIgnitionStatus/1

== system FusionMODEL_version1/SENSOR_MEASUREMENTS/RADAR_CAMERA_EGO_SENSOR_INTERFACE/RadarSensors ==
  time : Inport
  nObjRadar : Inport  Port=2
  RADSensorBUS : Inport  Port=3  OutDataTypeStr=Bus: RadarMeasParam  PortDimensions=200  BusOutputAsStruct=on
  Radar1 : Subsystem  TreatAsAtomicUnit=on
  Radar2 : Subsystem  TreatAsAtomicUnit=on
  Radar3 : Subsystem  TreatAsAtomicUnit=on
  Radar4 : Subsystem  TreatAsAtomicUnit=on
  Radar5 : Subsystem  TreatAsAtomicUnit=on
  Radar6 : Subsystem  TreatAsAtomicUnit=on
  R1 : Outport
  R2 : Outport  Port=2
  R3 : Outport  Port=3
  R4 : Outport  Port=4
  R5 : Outport  Port=5
  R6 : Outport  Port=6
  wires:
  RADSensorBUS/1 -> Radar2/3(SensorMeas), Radar6/3(SensorMeas), Radar5/3(SensorMeas), Radar4/3(SensorMeas), Radar3/3(SensorMeas), Radar1/3(SensorMeas)
  nObjRadar/1 -> Radar3/2(nObjRadar), Radar6/2(nObjRadar), Radar5/2(nObjRadar), Radar4/2(nObjRadar), Radar2/2(nObjRadar), Radar1/2(nObjRadar)
  Radar1/1(R1) -> R1/1
  time/1 -> Radar3/1(timeIdx), Radar6/1(timeIdx), Radar5/1(timeIdx), Radar4/1(timeIdx), Radar2/1(timeIdx), Radar1/1(timeIdx)
  Radar4/1(R4) -> R4/1
  Radar3/1(R3) -> R3/1
  Radar6/1(R6) -> R6/1
  Radar5/1(R5) -> R5/1
  Radar2/1(R2) -> R2/1

== system FusionMODEL_version1/SENSOR_MEASUREMENTS/RADAR_CAMERA_EGO_SENSOR_INTERFACE/RoadSensors ==
  time : Inport
  nLinesCamera : Inport  Port=2
  CameraLineCoeff1 : Inport  Port=3  OutDataTypeStr=Bus: LineMeasParam  PortDimensions=10
  Camera1 : Subsystem  TreatAsAtomicUnit=on
  Camera2 : Subsystem  TreatAsAtomicUnit=on
  Camera3 : Subsystem  TreatAsAtomicUnit=on
  Camera4 : Subsystem  TreatAsAtomicUnit=on
  Camera5 : Subsystem  TreatAsAtomicUnit=on
  Camera6 : Subsystem  TreatAsAtomicUnit=on
  Camera7 : Subsystem  TreatAsAtomicUnit=on
  Camera8 : Subsystem  TreatAsAtomicUnit=on
  C1 : Outport
  C2 : Outport  Port=2
  C3 : Outport  Port=3
  C4 : Outport  Port=4
  C5 : Outport  Port=5
  C6 : Outport  Port=6
  C7 : Outport  Port=7
  C8 : Outport  Port=8
  wires:
  Camera2/1(C1) -> C2/1
  Camera7/1(C1) -> C7/1
  CameraLineCoeff1/1 -> Camera1/3(CameraLineCoeff), Camera2/3(CameraLineCoeff), Camera3/3(CameraLineCoeff), Camera4/3(CameraLineCoeff), Camera5/3(CameraLineCoeff), Camera6/3(CameraLineCoeff), Camera8/3(CameraLineCoeff), Camera7/3(CameraLineCoeff)
  time/1 -> Camera1/1(timeIdx), Camera2/1(timeIdx), Camera3/1(timeIdx), Camera4/1(timeIdx), Camera5/1(timeIdx), Camera6/1(timeIdx), Camera8/1(timeIdx), Camera7/1(timeIdx)
  Camera1/1(C1) -> C1/1
  Camera6/1(C1) -> C6/1
  Camera5/1(C1) -> C5/1
  Camera8/1(C1) -> C8/1
  nLinesCamera/1 -> Camera2/2(nLines), Camera3/2(nLines), Camera4/2(nLines), Camera5/2(nLines), Camera6/2(nLines), Camera8/2(nLines), Camera7/2(nLines), Camera1/2(nLines)
  Camera3/1(C1) -> C3/1
  Camera4/1(C1) -> C4/1

== system FusionMODEL_version1/OBJECT_TRACKER_SENSOR_FUSION/SET_SENSOR_CALLIBRATION_PARAMETER/SET_CAMERA_SENSOR_PARAM/GET_DATA ==
  CAMSnsrParam : Inport
  Bus Selector : BusSelector  OutputSignals=CameraIntrinsics,CameraExtrinsics
  CameraIntrinsics : Outport
  CameraExtrinsics : Outport  Port=2
  wires:
  CAMSnsrParam/1 -> Bus Selector/1
  Bus Selector/2 -> CameraExtrinsics/1  "<CameraExtrinsics>"
  Bus Selector/1 -> CameraIntrinsics/1  "<CameraIntrinsics>"

== system FusionMODEL_version1/OBJECT_TRACKER_SENSOR_FUSION/SET_SENSOR_CALLIBRATION_PARAMETER/SET_CAMERA_SENSOR_PARAM/SET_CAMERA_EXTRINSIC_PARAM ==
  CameraCalibParam : Inport
  INSTALLED_CAMERA_i : ForIterator  IterationLimit=nCameras
  SET_CAMERA_EXTRINSIC_PARAM : Subsystem
  CameraCalibParamSet : Outport
  wires:
  INSTALLED_CAMERA_i/1 -> SET_CAMERA_EXTRINSIC_PARAM/2(SensorID)
  SET_CAMERA_EXTRINSIC_PARAM/1(Out1) -> CameraCalibParamSet/1
  CameraCalibParam/1 -> SET_CAMERA_EXTRINSIC_PARAM/1(SensorParam)

== system FusionMODEL_version1/OBJECT_TRACKER_SENSOR_FUSION/SET_SENSOR_CALLIBRATION_PARAMETER/SET_CAMERA_SENSOR_PARAM/SET_CAMERA_INTRINSIC_PARAM ==
  CameraCalibParam : Inport
  CAMERA_TYPE_i : ForIterator  IterationLimit=nCameraTypes
  SET_CAMERA_INTRINSIC_PARAM : Subsystem
  CameraCalibParamSet : Outport
  wires:
  CameraCalibParam/1 -> SET_CAMERA_INTRINSIC_PARAM/1(SensorParam)
  CAMERA_TYPE_i/1 -> SET_CAMERA_INTRINSIC_PARAM/2(SensorID)
  SET_CAMERA_INTRINSIC_PARAM/1(Out1) -> CameraCalibParamSet/1

== system FusionMODEL_version1/OBJECT_TRACKER_SENSOR_FUSION/SET_SENSOR_CALLIBRATION_PARAMETER/SET_CAMERA_SENSOR_PARAM/SET_DATA ==
  CameraIntrinsics : Inport
  CameraExtrinsics : Inport  Port=2
  Bus Creator : BusCreator  Inputs=2  OutDataTypeStr=Bus: CAM_SENSOR_PARAM  NonVirtualBus=on
  CAMSnsrParamUpd : Outport
  wires:
  Bus Creator/1 -> CAMSnsrParamUpd/1
  CameraIntrinsics/1 -> Bus Creator/1
  CameraExtrinsics/1 -> Bus Creator/2

== system FusionMODEL_version1/OBJECT_TRACKER_SENSOR_FUSION/SET_SENSOR_CALLIBRATION_PARAMETER/SET_RADAR_SENSOR_PARAM/GET_DATA ==
  RADSnsrParam : Inport
  Bus Selector : BusSelector  OutputSignals=RadarIntrinsics,RadarExtrinsics
  <RadarIntrinsics> : Outport
  <RadarExtrinsics> : Outport  Port=2
  wires:
  Bus Selector/1 -> <RadarIntrinsics>/1  "<RadarIntrinsics>"
  RADSnsrParam/1 -> Bus Selector/1
  Bus Selector/2 -> <RadarExtrinsics>/1  "<RadarExtrinsics>"

== system FusionMODEL_version1/OBJECT_TRACKER_SENSOR_FUSION/SET_SENSOR_CALLIBRATION_PARAMETER/SET_RADAR_SENSOR_PARAM/SET_DATA ==
  RadarIntrinsics : Inport
  RadarExtrinsics : Inport  Port=2
  Bus Creator : BusCreator  Inputs=2  OutDataTypeStr=Bus: RAD_SENSOR_PARAM  NonVirtualBus=on
  RADSnsrParamUpd : Outport
  wires:
  Bus Creator/1 -> RADSnsrParamUpd/1
  RadarIntrinsics/1 -> Bus Creator/1  "RadarIntrinsics"
  RadarExtrinsics/1 -> Bus Creator/2  "RadarExtrinsics"

== system FusionMODEL_version1/OBJECT_TRACKER_SENSOR_FUSION/SET_SENSOR_CALLIBRATION_PARAMETER/SET_RADAR_SENSOR_PARAM/SET_RADAR_EXTRINSIC_PARAM ==
  RadarCalibParam : Inport
  INSTALLED_RADAR_i : ForIterator  IterationLimit=nRadars
  SET_RADAR_EXTRINSIC_PARAM : Subsystem
  RadarCalibParamSet : Outport
  wires:
  RadarCalibParam/1 -> SET_RADAR_EXTRINSIC_PARAM/1(SensorParam)
  INSTALLED_RADAR_i/1 -> SET_RADAR_EXTRINSIC_PARAM/2(SensorID)
  SET_RADAR_EXTRINSIC_PARAM/1(RadarSensorParam) -> RadarCalibParamSet/1

== system FusionMODEL_version1/OBJECT_TRACKER_SENSOR_FUSION/SET_SENSOR_CALLIBRATION_PARAMETER/SET_RADAR_SENSOR_PARAM/SET_RADAR_INTRINSIC_PARAM ==
  RadarCalibParam : Inport
  RADAR_TYPE_i : ForIterator  IterationLimit=nRadarTypes
  SET_RADAR_INTRINSIC_PARAM : Subsystem
  RadarCalibParamSet : Outport
  wires:
  RadarCalibParam/1 -> SET_RADAR_INTRINSIC_PARAM/1(SensorParam)
  RADAR_TYPE_i/1 -> SET_RADAR_INTRINSIC_PARAM/2(SensorID)
  SET_RADAR_INTRINSIC_PARAM/1(RadarIntrinsicParam) -> RadarCalibParamSet/1

== system FusionMODEL_version1/OBJECT_TRACKER_SENSOR_FUSION/SPATIAL_ALLIGNMENT/CAMERA_MEASUREMENTS_SPATIAL_ALLIGNMENT/For Iterator Subsystem ==
  CameraCallibrationParam : Inport
  RadarStartingIdx : Inport  Port=2
  C1 : Inport  Port=3
  C2 : Inport  Port=4
  C3 : Inport  Port=5
  C4 : Inport  Port=6
  C5 : Inport  Port=7
  C6 : Inport  Port=8
  C7 : Inport  Port=9
  C8 : Inport  Port=10
  For Iterator : ForIterator  ResetStates=reset  IterationLimit=nCameras
  For Iterator Subsystem : Subsystem  TreatAsAtomicUnit=on
  InformationExtraction : Subsystem
  Subsystem : Subsystem
  MaxNoValidMeas : Outport
  CameraMeasTransformed : Outport  Port=2
  CameraMeasCOVTransformed : Outport  Port=3
  CameraMeasRef : Outport  Port=4
  wires:
  CameraCallibrationParam/1 -> InformationExtraction/1(CameraCallibration)
  C1/1 -> InformationExtraction/3(C1)
  C2/1 -> InformationExtraction/4(C2)
  C3/1 -> InformationExtraction/5(C3)
  C4/1 -> InformationExtraction/6(C4)
  C5/1 -> InformationExtraction/7(C5)
  C6/1 -> InformationExtraction/8(C6)
  InformationExtraction/1(CameraCalib) -> For Iterator Subsystem/1(CameraCalibration)
  InformationExtraction/2(nCameraMeas) -> For Iterator Subsystem/2(nMeas)
  InformationExtraction/3(CameraCANBus) -> For Iterator Subsystem/3(CameraCAN)
  RadarStartingIdx/1 -> InformationExtraction/11(StartingIndexes)
  Subsystem/1(nValidMeasVector) -> MaxNoValidMeas/1, Subsystem/1(nValidMeasVectorIn)
  InformationExtraction/4(MeasStartingIdx) -> Subsystem/7(StartIdx)
  C7/1 -> InformationExtraction/9(C7)
  C8/1 -> InformationExtraction/10(C8)
  For Iterator/1 -> Subsystem/2(SnsrIndex), InformationExtraction/2(CameraID)
  For Iterator Subsystem/1(nValidMeas) -> Subsystem/3(nValidMeas)
  For Iterator Subsystem/2(CameraMeasUpd) -> Subsystem/4(CameraCTSMeas)
  For Iterator Subsystem/3(CameraMeasNoiseCovUpd) -> Subsystem/5(CameraCTSNoiseCOV)
  For Iterator Subsystem/4(CameraMeasRefUpd) -> Subsystem/6(CameraCTSRef)
  Subsystem/2(CTSMat) -> CameraMeasTransformed/1, Subsystem/8(CTSMeasAllSensors)
  Subsystem/4(CTSMatRef) -> Subsystem/10(CTSRef), CameraMeasRef/1
  Subsystem/3(CTSMatNoiseCOV) -> CameraMeasCOVTransformed/1, Subsystem/9(CTSNoiseCOV)

== system FusionMODEL_version1/OBJECT_TRACKER_SENSOR_FUSION/SPATIAL_ALLIGNMENT/CAMERA_MEASUREMENTS_SPATIAL_ALLIGNMENT/RadarMeasurementIndexes2 ==
  validMeasCount : Inport
  CTSmeasMAT : Inport  Port=2
  CTSCovMAT : Inport  Port=3
  CTSRefMAT : Inport  Port=4
  Add{,1..6} (7 alike) : Sum
  Assignment1 : Assignment  NumberOfDimensions=2  DiagnosticForDimensions=Warning  IndexOptions=Assign all,Starting index (dialog)  Indices=1,1  OutputSizes=1,1
  Assignment2 : Assignment  NumberOfDimensions=3  DiagnosticForDimensions=Warning  IndexOptions=Assign all,Assign all,Starting index (dialog)  Indices=1,1,1  OutputSizes=1,1,1
  Assignment3 : Assignment  NumberOfDimensions=2  DiagnosticForDimensions=Warning  IndexOptions=Assign all,Starting index (dialog)  Indices=1,1  OutputSizes=1,1
  Bus Creator1 : BusCreator  Inputs=5  OutDataTypeStr=Bus: CAM_MEAS_MAT_CTS  NonVirtualBus=on
  Find Nonzero Elements1 : Find  NumberOfInputDimensions=3
  Mux1 : Mux  Inputs=8
  Reshape1 : Reshape  OutputDimensionality=Row vector (2-D)
  Selector : Selector  NumberOfDimensions=2  InputPortWidth=3  IndexOptions=Select all,Index vector (dialog)  Indices=1,1  OutputSizes=1,1
  Selector1 : Selector  NumberOfDimensions=2  InputPortWidth=3  IndexOptions=Select all,Index vector (dialog)  Indices=6,7  OutputSizes=1,1
  Selector11 : Selector  NumberOfDimensions=2  InputPortWidth=3  IndexOptions=Index vector (dialog),Select all  Indices=1,1  OutputSizes=1,1
  Selector12 : Selector  NumberOfDimensions=2  InputPortWidth=3  IndexOptions=Select all,Index vector (port)  Indices=1,1  OutputSizes=1,1
  Selector14 : Selector  NumberOfDimensions=2  InputPortWidth=3  IndexOptions=Select all,Index vector (port)  Indices=1,1  OutputSizes=1,1
  Selector15 : Selector  NumberOfDimensions=3  InputPortWidth=3  IndexOptions=Select all,Select all,Index vector (port)  Indices=1,1,1  OutputSizes=1,1,1
  Selector2 : Selector  NumberOfDimensions=2  InputPortWidth=3  IndexOptions=Select all,Index vector (dialog)  Indices=5,2  OutputSizes=1,1
  Selector3 : Selector  NumberOfDimensions=2  InputPortWidth=3  IndexOptions=Select all,Index vector (dialog)  Indices=5,3  OutputSizes=1,1
  Selector4 : Selector  NumberOfDimensions=2  InputPortWidth=3  IndexOptions=Select all,Index vector (dialog)  Indices=5,5  OutputSizes=1,1
  Selector5 : Selector  NumberOfDimensions=2  InputPortWidth=3  IndexOptions=Select all,Index vector (dialog)  Indices=6,6  OutputSizes=1,1
  Selector6 : Selector  NumberOfDimensions=2  InputPortWidth=3  IndexOptions=Select all,Index vector (dialog)  Indices=6,8  OutputSizes=1,1
  Selector8 : Selector  NumberOfDimensions=2  InputPortWidth=3  IndexOptions=Select all,Index vector (dialog)  Indices=5,4  OutputSizes=1,1
  CTSmeasMATout : Outport
  wires:
  validMeasCount/1 -> Selector2/1, Selector/1, Bus Creator1/4, Selector3/1, Selector6/1, Selector1/1, Selector5/1, Selector4/1, Selector8/1  "ValidMeasCountMeasCount"
  Add3/1 -> Add4/1, Mux1/5
  Selector3/1 -> Add1/2
  Add2/1 -> Add3/1, Mux1/4
  Add1/1 -> Mux1/3, Add2/1
  Selector4/1 -> Add3/2
  Selector/1 -> Mux1/1, Add/1
  Add/1 -> Add1/1, Mux1/2
  Add4/1 -> Add5/1, Mux1/6
  Selector2/1 -> Add/2
  Selector8/1 -> Add2/2
  Mux1/1 -> Reshape1/1
  Selector5/1 -> Add4/2
  Bus Creator1/1 -> CTSmeasMATout/1
  CTSRefMAT/1 -> [Ref], Selector11/1
  Selector11/1 -> Find Nonzero Elements1/1
  Find Nonzero Elements1/1 -> Selector14/2, Selector12/2, Selector15/2
  CTSmeasMAT/1 -> Assignment1/1, Selector14/1
  Selector14/1 -> Assignment1/2
  Selector15/1 -> Assignment2/2
  Selector12/1 -> Assignment3/2
  CTSCovMAT/1 -> Assignment2/1, Selector15/1
  Assignment3/1 -> Bus Creator1/3  "MeasRef"
  Assignment2/1 -> Bus Creator1/2  "MeasCovariance"
  Assignment1/1 -> Bus Creator1/1  "MeasArray"
  [Ref] -> Assignment3/1, Selector12/1
  Reshape1/1 -> Bus Creator1/5  "ValidCumulativeMeasCount"
  Add5/1 -> Add6/1, Mux1/7
  Selector1/1 -> Add5/2
  Add6/1 -> Mux1/8
  Selector6/1 -> Add6/2

== system FusionMODEL_version1/OBJECT_TRACKER_SENSOR_FUSION/SPATIAL_ALLIGNMENT/CAMERA_MEASUREMENTS_SPATIAL_ALLIGNMENT/StartingIndexes1 ==
  SnsrCallib : Inport
  CallibrationInfoExtractor : Subsystem
  Subsystem : Subsystem
  StartingIndexes : Outport
  wires:
  CallibrationInfoExtractor/1(C1nMeas) -> Subsystem/1(C1nMeas)
  CallibrationInfoExtractor/2(C2nMeas) -> Subsystem/2(C2nMeas)
  CallibrationInfoExtractor/3(C3nMeas) -> Subsystem/3(C3nMeas)
  CallibrationInfoExtractor/4(C4nMeas) -> Subsystem/4(C4nMeas)
  CallibrationInfoExtractor/5(C5nMeas) -> Subsystem/5(C5nMeas)
  Subsystem/1(StartingIndexes) -> StartingIndexes/1
  SnsrCallib/1 -> CallibrationInfoExtractor/1(SnsrCallib)
  CallibrationInfoExtractor/6(C6nMeas) -> Subsystem/6(C6nMeas)
  CallibrationInfoExtractor/7(C7nMeas) -> Subsystem/7(C7nMeas)

== system FusionMODEL_version1/OBJECT_TRACKER_SENSOR_FUSION/SPATIAL_ALLIGNMENT/RADAR_MEASUREMENTS_SPATIAL_ALLIGNMENT/RADAR_MEASUREMENTS_SPATIAL_ALLIGNMENT ==
  RadarCallibrationParam : Inport
  RadarStartingIdx : Inport  Port=2
  R1 : Inport  Port=3
  R2 : Inport  Port=4
  R3 : Inport  Port=5
  R4 : Inport  Port=6
  R5 : Inport  Port=7
  R6 : Inport  Port=8
  COORDINATE_TRANSFORMATION : Subsystem  TreatAsAtomicUnit=on
  GET_DATA : Subsystem
  SENSOR_LOOP : ForIterator  ResetStates=reset  IterationLimit=nRadars
  SET_DATA : Subsystem
  RadarMeasTransformed : Outport
  RadarMeasCOVTransformed : Outport  Port=2
  RadarMeasRef : Outport  Port=3
  MaxNoValidMeas : Outport  Port=4
  wires:
  RadarCallibrationParam/1 -> GET_DATA/1(RadarCallibration)
  R1/1 -> GET_DATA/3(R1)
  R2/1 -> GET_DATA/4(R2)
  R3/1 -> GET_DATA/5(R3)
  R4/1 -> GET_DATA/6(R4)
  R5/1 -> GET_DATA/7(R5)
  R6/1 -> GET_DATA/8(R6)
  GET_DATA/1(RadarCalib) -> COORDINATE_TRANSFORMATION/1(RadarCalibration)
  GET_DATA/2(nRadarMeas) -> COORDINATE_TRANSFORMATION/2(nMeas)
  GET_DATA/3(RadarCANBus) -> COORDINATE_TRANSFORMATION/3(RadarCAN)
  RadarStartingIdx/1 -> GET_DATA/9(StartingIndexes)
  SENSOR_LOOP/1 -> SET_DATA/2(SnsrIndex), GET_DATA/2(RadarID)
  SET_DATA/1(nValidMeasVector) -> SET_DATA/1(nValidMeasVectorIn), MaxNoValidMeas/1
  GET_DATA/4(MeasStartingIdx) -> SET_DATA/7(StartIdx)
  COORDINATE_TRANSFORMATION/1(nValidMeas) -> SET_DATA/3(nValidMeas)
  COORDINATE_TRANSFORMATION/2(RadarMeasUpd) -> SET_DATA/4(RadarCTSMeas)
  SET_DATA/2(CTSMat) -> SET_DATA/8(CTSMeasAllSensors), RadarMeasTransformed/1
  COORDINATE_TRANSFORMATION/3(RadarMeasNoiseCovUpd) -> SET_DATA/5(RadarCTSNoiseCOV)
  COORDINATE_TRANSFORMATION/4(RadarMeasRefUpd) -> SET_DATA/6(RadarCTSRef)
  SET_DATA/4(CTSMatRef) -> RadarMeasRef/1, SET_DATA/10(CTSRef)
  SET_DATA/3(CTSMatNoiseCOV) -> RadarMeasCOVTransformed/1, SET_DATA/9(CTSNoiseCOV)
